simulink model "linearizeDrone_umechTostate"  (R2015a)
settings: Solver=ode45  StartTime=0.0  StopTime=10.0  RelTol=1e-3
InitFcn:
  | % load parameters of the default quadrotor
  | disp('Quadrotor parameters loaded by InitFcn')
  | paramsFilters %load mdl_quadcopter as well!
undefined symbols (not defined in the file or in its folder): controlParams, quad
settings Model: Creator=ra  LastModifiedBy=ra

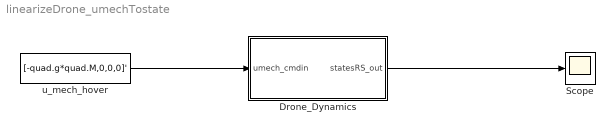
== system linearizeDrone_umechTostate ==
  Drone_Dynamics : Subsystem
  Scope : Scope
  u_mech_hover : Constant  Value=[-quad.g*quad.M,0,0,0]'
  wires:
  u_mech_hover/1 -> Drone_Dynamics/1(umech_cmdin)
  Drone_Dynamics/1(statesRS_out) -> Scope/1

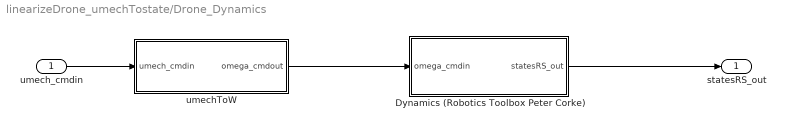
== system linearizeDrone_umechTostate/Drone_Dynamics ==
  umech_cmdin : Inport
  Dynamics (Robotics Toolbox Peter Corke) : Subsystem
  umechToW : Subsystem
  statesRS_out : Outport
  wires:
  umech_cmdin/1 -> umechToW/1(umech_cmdin)
  umechToW/1(omega_cmdout) -> Dynamics (Robotics Toolbox Peter Corke)/1(omega_cmdin)
  Dynamics (Robotics Toolbox Peter Corke)/1(statesRS_out) -> statesRS_out/1

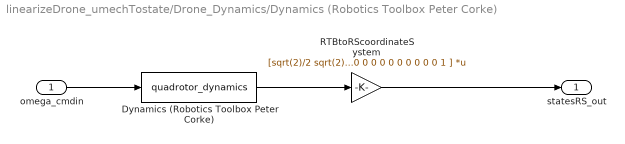
== system linearizeDrone_umechTostate/Drone_Dynamics/Dynamics (Robotics Toolbox Peter Corke) ==
  omega_cmdin : Inport
  Dynamics (Robotics Toolbox Peter Corke) : S-Function  FunctionName=quadrotor_dynamics  Parameters=quad
  RTBtoRScoordinateSystem : Gain  Gain=|  Multiplication=Matrix(K*u)
      | [sqrt(2)/2 sqrt(2)/2 0 0 0 0 0 0 0 0 0 0;
      |  -sqrt(2)/2 sqrt(2)/2  0 0 0 0 0 0 0 0 0 0;   
      |  0 0 1 0 0 0 0 0 0 0 0 0;
      |  0 0 0 1 0 0 0 0 0 0 0 0;
      |  0 0 0 0 sqrt(2)/2 -sqrt(2)/2 0 0 0 0 0 0;
      |  0 0 0 0 sqrt(2)/2 sqrt(2)/2  0 0 0 0 0 0;    
      |  0 0 0 0 0 0 sqrt(2)/2 sqrt(2)/2 0 0 0 0 ;
      |  0 0 0 0 0 0 -sqrt(2)/2 sqrt(2)/2  0 0 0 0 ;   
      |  0 0 0 0 0 0 0 0 1 0 0 0;
      |  0 0 0 0 0 0 0 0 0 sqrt(2)/2 -sqrt(2)/2 0;
      |  0 0 0 0 0 0 0 0 0 sqrt(2)/2 sqrt(2)/2 0;
      |  0 0 0 0 0 0 0 0 0 0 0 1
      | ]
  statesRS_out : Outport
  wires:
  Dynamics (Robotics Toolbox Peter Corke)/1 -> RTBtoRScoordinateSystem/1
  RTBtoRScoordinateSystem/1 -> statesRS_out/1
  omega_cmdin/1 -> Dynamics (Robotics Toolbox Peter Corke)/1

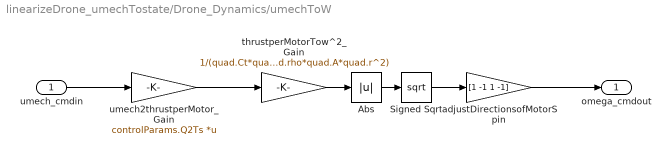
== system linearizeDrone_umechTostate/Drone_Dynamics/umechToW ==
  umech_cmdin : Inport
  Abs : Abs
  Signed Sqrt : Sqrt  SaturateOnIntegerOverflow=on
  adjustDirectionsofMotorSpin : Gain  Gain=[1 -1 1 -1]
  thrustperMotorTow^2_Gain : Gain  Gain=1/(quad.Ct*quad.rho*quad.A*quad.r^2)
  umech2thrustperMotor_Gain : Gain  Gain=controlParams.Q2Ts  Multiplication=Matrix(K*u)
  omega_cmdout : Outport
  wires:
  umech2thrustperMotor_Gain/1 -> thrustperMotorTow^2_Gain/1
  umech_cmdin/1 -> umech2thrustperMotor_Gain/1
  Signed Sqrt/1 -> adjustDirectionsofMotorSpin/1
  thrustperMotorTow^2_Gain/1 -> Abs/1
  adjustDirectionsofMotorSpin/1 -> omega_cmdout/1
  Abs/1 -> Signed Sqrt/1
